simulink model "draft7"  (R2023a)
settings: Solver=VariableStepAuto  StartTime=0.0  StopTime=10  FixedStep=0.0001  MaxStep=0.1  RelTol=1e-3  AbsTol=1e-3  EnableMultiTasking=on
model workspace (MAT data in the model file):
  C_Gimbal = 0.1
  C_IAP = 0.01
  IAP_Pa = 0
  K_Gimbal = 0
  K_IAP = 10
  LeftAbdominalMuscleForce = 0
  LeftBackMuscleForce = 0
  LeftTransverse1MuscleForce = 0
  LeftTransverse2MuscleForce = 0
  Moment_AR = 0
  Moment_FE = 0
  Moment_LB = 0
  RightAbdominalMuscleForce = 0
  RightBackMuscleForce = 0
  RightTransverse1MuscleForce = 0
  RightTransverse2MuscleForce = 0
  a = 1
  b = 1
undefined symbols (not defined in the file): X, Y, Z
libraries: sm_lib x279, nesl_utility x233, simulink_extras x33, checkpacklib x3, simulink x1
(part 7 of 7)

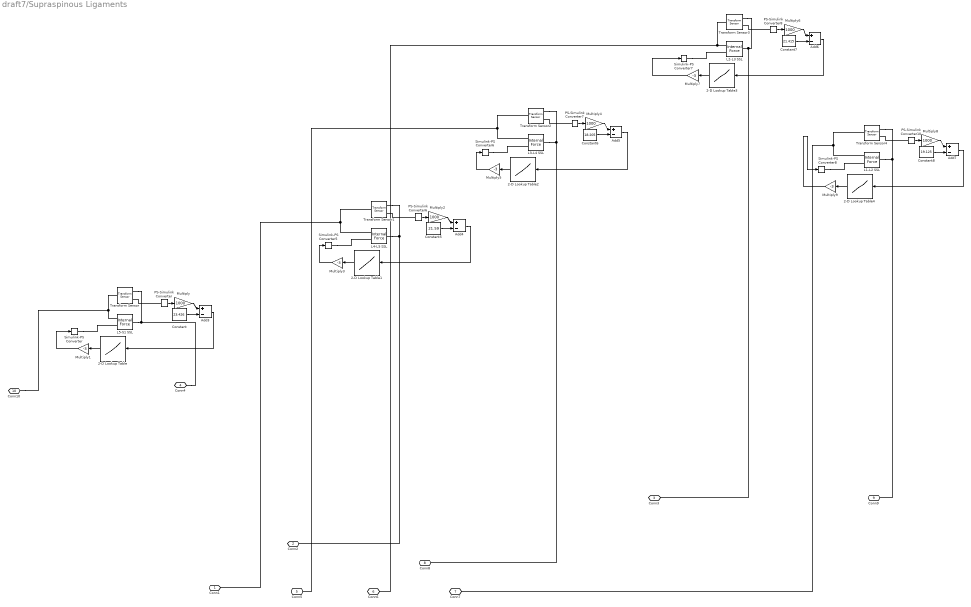
== system draft7/Supraspinous Ligaments ==
  2-D Lookup Table : Lookup_n-D  NumberOfTableDimensions=1  BreakpointsForDimension1=[0;0.272;4.08;5.984;7.888]  BreakpointsForDimension2=[1:3]  Table=[0;0;8.4;21;84]  InternalRulePriority=Speed  RndMeth=Simplest
  2-D Lookup Table1 : Lookup_n-D  NumberOfTableDimensions=1  BreakpointsForDimension1=[0;0.223;3.345;4.906;6.467]  BreakpointsForDimension2=[1:3]  Table=[0;0;8.4;21;84]  InternalRulePriority=Speed  RndMeth=Simplest
  2-D Lookup Table2 : Lookup_n-D  NumberOfTableDimensions=1  BreakpointsForDimension1=[0;0.194;2.91;4.268;5.626]  BreakpointsForDimension2=[1:3]  Table=[0;0;8.4;21;84]  InternalRulePriority=Speed  RndMeth=Simplest
  2-D Lookup Table3 : Lookup_n-D  NumberOfTableDimensions=1  BreakpointsForDimension1=[0;0.268;4.02;5.896;7.772]  BreakpointsForDimension2=[1:3]  Table=[0;0;8.4;21;84]  InternalRulePriority=Speed  RndMeth=Simplest
  2-D Lookup Table4 : Lookup_n-D  NumberOfTableDimensions=1  BreakpointsForDimension1=[0;0.223;3.345;4.906;6.467]  BreakpointsForDimension2=[1:3]  Table=[0;0;8.4;21;84]  InternalRulePriority=Speed  RndMeth=Simplest
  Add{3..7} (5 alike) : Sum  Inputs=+-
  Constant : Constant  Value=23.426
  Constant5 : Constant  Value=21.59
  Constant6 : Constant  Value=18.205
  Constant7 : Constant  Value=21.415
  Constant8 : Constant  Value=19.125
  L1-L2 SSL : sm_lib/Forces and Torques/Internal Force
  L2-L3 SSL : sm_lib/Forces and Torques/Internal Force
  L3-L4 SSL : sm_lib/Forces and Torques/Internal Force
  L4-L5 SSL : sm_lib/Forces and Torques/Internal Force
  L5-S1 SSL : sm_lib/Forces and Torques/Internal Force
  Multiply{,2,4,6,8} (5 alike) : Gain  Gain=1000
  Multiply{1,3,5,7,9} (5 alike) : Gain  Gain=-3
  PS-Simulink Converter{,6..8,10} (5 alike) : nesl_utility/PS-Simulink Converter  PhysicalDomain=network_engine_domain  SubClassName=ps_output  LeftPortType=input  RightPortType=output  PseudoPeriodic=off  Frequencies=[]  VectorFormat=inherit  Unit=inherit  AffineConversion=off
  Simulink-PS Converter{,5..8} (5 alike) : nesl_utility/Simulink-PS Converter  PhysicalDomain=network_engine_domain  SubClassName=ps_input  LeftPortType=input  RightPortType=output  PseudoPeriodic=off  Frequencies=[]  NoiseDistribution=none  NoiseParameters=[]  Unit=1  AffineConversion=off  FilteringAndDerivatives=provide  SimscapeFilterOrder=1  InputFilterTimeConstant=0.001  UdotUserProvided=0
  Transform Sensor{,1..4} (5 alike) : sm_lib/Frames and Transforms/Transform Sensor  MeasurementFrame=World  RotationSequence=XYX  SenseAngle=off  SenseAxis=off  SenseQ=off  SenseR=off  SenseRotationSequence=off  SenseOmegaX=off  SenseOmegaY=off  SenseOmegaZ=off  SenseQDot=off  SenseRDot=off  SenseRotationSequenceDot=off  SenseAlphaX=off  SenseAlphaY=off  SenseAlphaZ=off  SenseQDDot=off  SenseRDDot=off  SenseX=off  SenseY=off  SenseZ=off  SenseRad=off  SenseAzim=off  SenseDist=on  SenseInc=off  SenseXDot=off  SenseYDot=off  SenseZDot=off  SenseRadDot=off  SenseAzimDot=off  SenseDistDot=off  SenseIncDot=off  SenseXDDot=off  SenseYDDot=off  SenseZDDot=off  SenseRadDDot=off  SenseAzimDDot=off  SenseDistDDot=off  SenseIncDDot=off
  Conn1 : PMIOPort  Side=Left
  Conn2 : PMIOPort  Port=2  Side=Left
  Conn3 : PMIOPort  Port=3  Side=Left
  Conn4 : PMIOPort  Port=4  Side=Left
  Conn5 : PMIOPort  Port=5  Side=Left
  Conn6 : PMIOPort  Port=6  Side=Left
  Conn7 : PMIOPort  Port=7  Side=Left
  Conn8 : PMIOPort  Port=8  Side=Left
  Conn9 : PMIOPort  Port=9  Side=Left
  Conn10 : PMIOPort  Port=10  Side=Left
  wires:
  Constant6/1 -> Add5/2
  Add6/1 -> 2-D Lookup Table3/1
  PS-Simulink Converter10/1 -> Multiply8/1
  Add4/1 -> 2-D Lookup Table1/1
  Multiply1/1 -> Simulink-PS Converter/1
  Multiply/1 -> Add3/1
  Multiply7/1 -> Simulink-PS Converter7/1
  Multiply8/1 -> Add7/1
  2-D Lookup Table3/1 -> Multiply7/1
  Multiply6/1 -> Add6/1
  Add3/1 -> 2-D Lookup Table/1
  2-D Lookup Table2/1 -> Multiply5/1
  Constant5/1 -> Add4/2
  PS-Simulink Converter/1 -> Multiply/1
  Constant/1 -> Add3/2
  2-D Lookup Table/1 -> Multiply1/1
  2-D Lookup Table4/1 -> Multiply9/1
  Multiply2/1 -> Add4/1
  Add7/1 -> 2-D Lookup Table4/1
  Multiply3/1 -> Simulink-PS Converter5/1
  Add5/1 -> 2-D Lookup Table2/1
  PS-Simulink Converter8/1 -> Multiply6/1
  Constant7/1 -> Add6/2
  Multiply9/1 -> Simulink-PS Converter8/1
  Constant8/1 -> Add7/2
  2-D Lookup Table1/1 -> Multiply3/1
  Multiply5/1 -> Simulink-PS Converter6/1
  PS-Simulink Converter6/1 -> Multiply2/1
  Multiply4/1 -> Add5/1
  PS-Simulink Converter7/1 -> Multiply4/1
  connections:
  L5-S1 SSL/LConn1 -- Conn10/RConn1 -- Transform Sensor/LConn1
  Simulink-PS Converter8/RConn1 -- L1-L2 SSL/LConn2
  L4-L5 SSL/LConn1 -- Conn1/RConn1 -- Transform Sensor1/LConn1
  L1-L2 SSL/LConn1 -- Conn7/RConn1 -- Transform Sensor4/LConn1
  Simulink-PS Converter/RConn1 -- L5-S1 SSL/LConn2
  PS-Simulink Converter6/LConn1 -- Transform Sensor1/RConn2
  L4-L5 SSL/RConn1 -- Transform Sensor1/RConn1 -- Conn2/RConn1
  PS-Simulink Converter/LConn1 -- Transform Sensor/RConn2
  L5-S1 SSL/RConn1 -- Conn4/RConn1 -- Transform Sensor/RConn1
  L3-L4 SSL/LConn1 -- Conn5/RConn1 -- Transform Sensor2/LConn1
  PS-Simulink Converter8/LConn1 -- Transform Sensor3/RConn2
  PS-Simulink Converter10/LConn1 -- Transform Sensor4/RConn2
  L2-L3 SSL/RConn1 -- Conn3/RConn1 -- Transform Sensor3/RConn1
  PS-Simulink Converter7/LConn1 -- Transform Sensor2/RConn2
  L1-L2 SSL/RConn1 -- Conn9/RConn1 -- Transform Sensor4/RConn1
  L2-L3 SSL/LConn1 -- Conn6/RConn1 -- Transform Sensor3/LConn1
  Transform Sensor2/RConn1 -- Conn8/RConn1 -- L3-L4 SSL/RConn1
  Simulink-PS Converter7/RConn1 -- L2-L3 SSL/LConn2
  Simulink-PS Converter5/RConn1 -- L4-L5 SSL/LConn2
  Simulink-PS Converter6/RConn1 -- L3-L4 SSL/LConn2

== system draft7/L1/AR torque feedback L4 ==
  Constant : Constant  Value=0.7
  Constant1 : Constant  Value=0.7
  Gain5 : Gain  Gain=-1
  PS-Simulink Converter9 : nesl_utility/PS-Simulink Converter  PhysicalDomain=network_engine_domain  SubClassName=ps_output  LeftPortType=input  RightPortType=output  PseudoPeriodic=off  Frequencies=[]  VectorFormat=1-D array  Unit=inherit  AffineConversion=off
  Radians to Degrees : simulink_extras/Transformations/Radians to Degrees
  Simulink-PS Converter6 : nesl_utility/Simulink-PS Converter  PhysicalDomain=network_engine_domain  SubClassName=ps_input  LeftPortType=input  RightPortType=output  PseudoPeriodic=off  Frequencies=[]  NoiseDistribution=none  NoiseParameters=[]  Unit=1  AffineConversion=off  FilteringAndDerivatives=provide  SimscapeFilterOrder=1  InputFilterTimeConstant=0.001  UdotUserProvided=0
  peacewise torque profile5 : MATLAB Function  TreatAsAtomicUnit=on
  AR rot : PMIOPort  Side=Left
  AR torque : PMIOPort  Port=2  Side=Right
  wires:
  PS-Simulink Converter9/1 -> Radians to Degrees/1
  peacewise torque profile5/1(torque) -> Gain5/1
  Gain5/1 -> Simulink-PS Converter6/1
  Radians to Degrees/1 -> peacewise torque profile5/1(u)
  Constant/1 -> peacewise torque profile5/2(a)
  Constant1/1 -> peacewise torque profile5/3(b)
  connections:
  PS-Simulink Converter9/LConn1 -- AR rot/RConn1
  AR torque/RConn1 -- Simulink-PS Converter6/RConn1

== system draft7/L1/FE torque feedback L4 ==
  Constant : Constant  Value=a
  Constant1 : Constant  Value=b
  Gain1 : Gain  Gain=-1
  Gain7 : Gain
  PS-Simulink Converter5 : nesl_utility/PS-Simulink Converter  PhysicalDomain=network_engine_domain  SubClassName=ps_output  LeftPortType=input  RightPortType=output  PseudoPeriodic=off  Frequencies=[]  VectorFormat=1-D array  Unit=inherit  AffineConversion=off
  Radians to Degrees : simulink_extras/Transformations/Radians to Degrees
  Simulink-PS Converter4 : nesl_utility/Simulink-PS Converter  PhysicalDomain=network_engine_domain  SubClassName=ps_input  LeftPortType=input  RightPortType=output  PseudoPeriodic=off  Frequencies=[]  NoiseDistribution=none  NoiseParameters=[]  Unit=1  AffineConversion=off  FilteringAndDerivatives=provide  SimscapeFilterOrder=1  InputFilterTimeConstant=0.001  UdotUserProvided=0
  peacewise torque profile1 : MATLAB Function  TreatAsAtomicUnit=on
  FE rot : PMIOPort  Side=Left
  FE torque : PMIOPort  Port=2  Side=Right
  wires:
  PS-Simulink Converter5/1 -> Radians to Degrees/1
  peacewise torque profile1/1(torque) -> Gain7/1
  Gain7/1 -> Simulink-PS Converter4/1
  Radians to Degrees/1 -> Gain1/1
  Gain1/1 -> peacewise torque profile1/1(u)
  Constant/1 -> peacewise torque profile1/2(a)
  Constant1/1 -> peacewise torque profile1/3(b)
  connections:
  FE rot/RConn1 -- PS-Simulink Converter5/LConn1
  FE torque/RConn1 -- Simulink-PS Converter4/RConn1

== system draft7/L1/LB torque feedback L4 ==
  Constant : Constant  Value=a
  Constant1 : Constant  Value=b
  Gain4 : Gain  Gain=-1
  PS-Simulink Converter8 : nesl_utility/PS-Simulink Converter  PhysicalDomain=network_engine_domain  SubClassName=ps_output  LeftPortType=input  RightPortType=output  PseudoPeriodic=off  Frequencies=[]  VectorFormat=1-D array  Unit=inherit  AffineConversion=off
  Radians to Degrees : simulink_extras/Transformations/Radians to Degrees
  Simulink-PS Converter5 : nesl_utility/Simulink-PS Converter  PhysicalDomain=network_engine_domain  SubClassName=ps_input  LeftPortType=input  RightPortType=output  PseudoPeriodic=off  Frequencies=[]  NoiseDistribution=none  NoiseParameters=[]  Unit=1  AffineConversion=off  FilteringAndDerivatives=provide  SimscapeFilterOrder=1  InputFilterTimeConstant=0.001  UdotUserProvided=0
  peacewise torque profile4 : MATLAB Function  TreatAsAtomicUnit=on
  LB rot : PMIOPort  Side=Left
  LB torque : PMIOPort  Port=2  Side=Right
  wires:
  Gain4/1 -> Simulink-PS Converter5/1
  PS-Simulink Converter8/1 -> Radians to Degrees/1
  peacewise torque profile4/1(torque) -> Gain4/1
  Constant/1 -> peacewise torque profile4/2(a)
  Constant1/1 -> peacewise torque profile4/3(b)
  Radians to Degrees/1 -> peacewise torque profile4/1(u)
  connections:
  Simulink-PS Converter5/RConn1 -- LB torque/RConn1
  LB rot/RConn1 -- PS-Simulink Converter8/LConn1

== system draft7/L2/AR torque feedback L4 ==
  Constant : Constant  Value=0.7
  Constant1 : Constant  Value=0.7
  Gain5 : Gain  Gain=-1
  PS-Simulink Converter9 : nesl_utility/PS-Simulink Converter  PhysicalDomain=network_engine_domain  SubClassName=ps_output  LeftPortType=input  RightPortType=output  PseudoPeriodic=off  Frequencies=[]  VectorFormat=1-D array  Unit=inherit  AffineConversion=off
  Radians to Degrees : simulink_extras/Transformations/Radians to Degrees
  Simulink-PS Converter6 : nesl_utility/Simulink-PS Converter  PhysicalDomain=network_engine_domain  SubClassName=ps_input  LeftPortType=input  RightPortType=output  PseudoPeriodic=off  Frequencies=[]  NoiseDistribution=none  NoiseParameters=[]  Unit=1  AffineConversion=off  FilteringAndDerivatives=provide  SimscapeFilterOrder=1  InputFilterTimeConstant=0.001  UdotUserProvided=0
  peacewise torque profile5 : MATLAB Function  TreatAsAtomicUnit=on
  AR rot : PMIOPort  Side=Left
  AR torque : PMIOPort  Port=2  Side=Right
  wires:
  Gain5/1 -> Simulink-PS Converter6/1
  peacewise torque profile5/1(torque) -> Gain5/1
  PS-Simulink Converter9/1 -> Radians to Degrees/1
  Radians to Degrees/1 -> peacewise torque profile5/1(u)
  Constant/1 -> peacewise torque profile5/2(a)
  Constant1/1 -> peacewise torque profile5/3(b)
  connections:
  AR torque/RConn1 -- Simulink-PS Converter6/RConn1
  PS-Simulink Converter9/LConn1 -- AR rot/RConn1

== system draft7/L2/FE torque feedback L4 ==
  Constant : Constant  Value=a
  Constant1 : Constant  Value=b
  Gain1 : Gain  Gain=-1
  Gain7 : Gain
  PS-Simulink Converter5 : nesl_utility/PS-Simulink Converter  PhysicalDomain=network_engine_domain  SubClassName=ps_output  LeftPortType=input  RightPortType=output  PseudoPeriodic=off  Frequencies=[]  VectorFormat=1-D array  Unit=inherit  AffineConversion=off
  Radians to Degrees : simulink_extras/Transformations/Radians to Degrees
  Simulink-PS Converter4 : nesl_utility/Simulink-PS Converter  PhysicalDomain=network_engine_domain  SubClassName=ps_input  LeftPortType=input  RightPortType=output  PseudoPeriodic=off  Frequencies=[]  NoiseDistribution=none  NoiseParameters=[]  Unit=1  AffineConversion=off  FilteringAndDerivatives=provide  SimscapeFilterOrder=1  InputFilterTimeConstant=0.001  UdotUserProvided=0
  peacewise torque profile1 : MATLAB Function  TreatAsAtomicUnit=on
  FE rot : PMIOPort  Side=Left
  FE torque : PMIOPort  Port=2  Side=Right
  wires:
  Gain7/1 -> Simulink-PS Converter4/1
  peacewise torque profile1/1(torque) -> Gain7/1
  Radians to Degrees/1 -> Gain1/1
  PS-Simulink Converter5/1 -> Radians to Degrees/1
  Constant/1 -> peacewise torque profile1/2(a)
  Constant1/1 -> peacewise torque profile1/3(b)
  Gain1/1 -> peacewise torque profile1/1(u)
  connections:
  FE torque/RConn1 -- Simulink-PS Converter4/RConn1
  FE rot/RConn1 -- PS-Simulink Converter5/LConn1

== system draft7/L2/LB torque feedback L4 ==
  Constant : Constant  Value=a
  Constant1 : Constant  Value=b
  Gain4 : Gain  Gain=-1
  PS-Simulink Converter8 : nesl_utility/PS-Simulink Converter  PhysicalDomain=network_engine_domain  SubClassName=ps_output  LeftPortType=input  RightPortType=output  PseudoPeriodic=off  Frequencies=[]  VectorFormat=1-D array  Unit=inherit  AffineConversion=off
  Radians to Degrees : simulink_extras/Transformations/Radians to Degrees
  Simulink-PS Converter5 : nesl_utility/Simulink-PS Converter  PhysicalDomain=network_engine_domain  SubClassName=ps_input  LeftPortType=input  RightPortType=output  PseudoPeriodic=off  Frequencies=[]  NoiseDistribution=none  NoiseParameters=[]  Unit=1  AffineConversion=off  FilteringAndDerivatives=provide  SimscapeFilterOrder=1  InputFilterTimeConstant=0.001  UdotUserProvided=0
  peacewise torque profile4 : MATLAB Function  TreatAsAtomicUnit=on
  LB rot : PMIOPort  Side=Left
  LB torque : PMIOPort  Port=2  Side=Right
  wires:
  peacewise torque profile4/1(torque) -> Gain4/1
  PS-Simulink Converter8/1 -> Radians to Degrees/1
  Gain4/1 -> Simulink-PS Converter5/1
  Constant/1 -> peacewise torque profile4/2(a)
  Constant1/1 -> peacewise torque profile4/3(b)
  Radians to Degrees/1 -> peacewise torque profile4/1(u)
  connections:
  LB rot/RConn1 -- PS-Simulink Converter8/LConn1
  Simulink-PS Converter5/RConn1 -- LB torque/RConn1

== system draft7/L3/AR torque feedback L4 ==
  Constant : Constant  Value=0.7
  Constant1 : Constant  Value=0.7
  Gain5 : Gain  Gain=-1
  PS-Simulink Converter9 : nesl_utility/PS-Simulink Converter  PhysicalDomain=network_engine_domain  SubClassName=ps_output  LeftPortType=input  RightPortType=output  PseudoPeriodic=off  Frequencies=[]  VectorFormat=1-D array  Unit=inherit  AffineConversion=off
  Radians to Degrees : simulink_extras/Transformations/Radians to Degrees
  Simulink-PS Converter6 : nesl_utility/Simulink-PS Converter  PhysicalDomain=network_engine_domain  SubClassName=ps_input  LeftPortType=input  RightPortType=output  PseudoPeriodic=off  Frequencies=[]  NoiseDistribution=none  NoiseParameters=[]  Unit=1  AffineConversion=off  FilteringAndDerivatives=provide  SimscapeFilterOrder=1  InputFilterTimeConstant=0.001  UdotUserProvided=0
  peacewise torque profile5 : MATLAB Function  TreatAsAtomicUnit=on
  AR rot : PMIOPort  Side=Left
  AR torque : PMIOPort  Port=2  Side=Right
  wires:
  peacewise torque profile5/1(torque) -> Gain5/1
  Gain5/1 -> Simulink-PS Converter6/1
  PS-Simulink Converter9/1 -> Radians to Degrees/1
  Radians to Degrees/1 -> peacewise torque profile5/1(u)
  Constant/1 -> peacewise torque profile5/2(a)
  Constant1/1 -> peacewise torque profile5/3(b)
  connections:
  PS-Simulink Converter9/LConn1 -- AR rot/RConn1
  AR torque/RConn1 -- Simulink-PS Converter6/RConn1

== system draft7/L3/FE torque feedback L4 ==
  Constant : Constant  Value=a
  Constant1 : Constant  Value=b
  Gain1 : Gain  Gain=-1
  Gain7 : Gain
  PS-Simulink Converter5 : nesl_utility/PS-Simulink Converter  PhysicalDomain=network_engine_domain  SubClassName=ps_output  LeftPortType=input  RightPortType=output  PseudoPeriodic=off  Frequencies=[]  VectorFormat=1-D array  Unit=inherit  AffineConversion=off
  Radians to Degrees : simulink_extras/Transformations/Radians to Degrees
  Simulink-PS Converter4 : nesl_utility/Simulink-PS Converter  PhysicalDomain=network_engine_domain  SubClassName=ps_input  LeftPortType=input  RightPortType=output  PseudoPeriodic=off  Frequencies=[]  NoiseDistribution=none  NoiseParameters=[]  Unit=1  AffineConversion=off  FilteringAndDerivatives=provide  SimscapeFilterOrder=1  InputFilterTimeConstant=0.001  UdotUserProvided=0
  peacewise torque profile1 : MATLAB Function  TreatAsAtomicUnit=on
  FE rot : PMIOPort  Side=Left
  FE torque : PMIOPort  Port=2  Side=Right
  wires:
  peacewise torque profile1/1(torque) -> Gain7/1
  Gain7/1 -> Simulink-PS Converter4/1
  Radians to Degrees/1 -> Gain1/1
  PS-Simulink Converter5/1 -> Radians to Degrees/1
  Constant/1 -> peacewise torque profile1/2(a)
  Constant1/1 -> peacewise torque profile1/3(b)
  Gain1/1 -> peacewise torque profile1/1(u)
  connections:
  FE rot/RConn1 -- PS-Simulink Converter5/LConn1
  FE torque/RConn1 -- Simulink-PS Converter4/RConn1

== system draft7/L3/LB torque feedback L4 ==
  Constant : Constant  Value=a
  Constant1 : Constant  Value=b
  Gain4 : Gain  Gain=-1
  PS-Simulink Converter8 : nesl_utility/PS-Simulink Converter  PhysicalDomain=network_engine_domain  SubClassName=ps_output  LeftPortType=input  RightPortType=output  PseudoPeriodic=off  Frequencies=[]  VectorFormat=1-D array  Unit=inherit  AffineConversion=off
  Radians to Degrees : simulink_extras/Transformations/Radians to Degrees
  Simulink-PS Converter5 : nesl_utility/Simulink-PS Converter  PhysicalDomain=network_engine_domain  SubClassName=ps_input  LeftPortType=input  RightPortType=output  PseudoPeriodic=off  Frequencies=[]  NoiseDistribution=none  NoiseParameters=[]  Unit=1  AffineConversion=off  FilteringAndDerivatives=provide  SimscapeFilterOrder=1  InputFilterTimeConstant=0.001  UdotUserProvided=0
  peacewise torque profile4 : MATLAB Function  TreatAsAtomicUnit=on
  LB rot : PMIOPort  Side=Left
  LB torque : PMIOPort  Port=2  Side=Right
  wires:
  Gain4/1 -> Simulink-PS Converter5/1
  PS-Simulink Converter8/1 -> Radians to Degrees/1
  peacewise torque profile4/1(torque) -> Gain4/1
  Constant/1 -> peacewise torque profile4/2(a)
  Constant1/1 -> peacewise torque profile4/3(b)
  Radians to Degrees/1 -> peacewise torque profile4/1(u)
  connections:
  Simulink-PS Converter5/RConn1 -- LB torque/RConn1
  LB rot/RConn1 -- PS-Simulink Converter8/LConn1

== system draft7/L4/AR torque feedback L4 ==
  Constant : Constant  Value=0.7
  Constant1 : Constant  Value=0.7
  Gain5 : Gain  Gain=-1
  PS-Simulink Converter9 : nesl_utility/PS-Simulink Converter  PhysicalDomain=network_engine_domain  SubClassName=ps_output  LeftPortType=input  RightPortType=output  PseudoPeriodic=off  Frequencies=[]  VectorFormat=1-D array  Unit=inherit  AffineConversion=off
  Radians to Degrees : simulink_extras/Transformations/Radians to Degrees
  Simulink-PS Converter6 : nesl_utility/Simulink-PS Converter  PhysicalDomain=network_engine_domain  SubClassName=ps_input  LeftPortType=input  RightPortType=output  PseudoPeriodic=off  Frequencies=[]  NoiseDistribution=none  NoiseParameters=[]  Unit=1  AffineConversion=off  FilteringAndDerivatives=provide  SimscapeFilterOrder=1  InputFilterTimeConstant=0.001  UdotUserProvided=0
  peacewise torque profile5 : MATLAB Function  TreatAsAtomicUnit=on
  AR rot : PMIOPort  Side=Left
  AR torque : PMIOPort  Port=2  Side=Right
  wires:
  Gain5/1 -> Simulink-PS Converter6/1
  peacewise torque profile5/1(torque) -> Gain5/1
  PS-Simulink Converter9/1 -> Radians to Degrees/1
  Radians to Degrees/1 -> peacewise torque profile5/1(u)
  Constant/1 -> peacewise torque profile5/2(a)
  Constant1/1 -> peacewise torque profile5/3(b)
  connections:
  AR torque/RConn1 -- Simulink-PS Converter6/RConn1
  PS-Simulink Converter9/LConn1 -- AR rot/RConn1

== system draft7/L4/FE torque feedback L4 ==
  Constant : Constant  Value=a
  Constant1 : Constant  Value=b
  Gain1 : Gain  Gain=-1
  Gain7 : Gain
  PS-Simulink Converter5 : nesl_utility/PS-Simulink Converter  PhysicalDomain=network_engine_domain  SubClassName=ps_output  LeftPortType=input  RightPortType=output  PseudoPeriodic=off  Frequencies=[]  VectorFormat=1-D array  Unit=inherit  AffineConversion=off
  Radians to Degrees : simulink_extras/Transformations/Radians to Degrees
  Scope : Scope  NumInputPorts=2
  Simulink-PS Converter4 : nesl_utility/Simulink-PS Converter  PhysicalDomain=network_engine_domain  SubClassName=ps_input  LeftPortType=input  RightPortType=output  PseudoPeriodic=off  Frequencies=[]  NoiseDistribution=none  NoiseParameters=[]  Unit=1  AffineConversion=off  FilteringAndDerivatives=provide  SimscapeFilterOrder=1  InputFilterTimeConstant=0.001  UdotUserProvided=0
  peacewise torque profile1 : MATLAB Function  TreatAsAtomicUnit=on
  FE rot : PMIOPort  Side=Left
  FE torque : PMIOPort  Port=2  Side=Right
  wires:
  Gain7/1 -> Scope/2, Simulink-PS Converter4/1
  peacewise torque profile1/1(torque) -> Gain7/1
  Radians to Degrees/1 -> Gain1/1
  PS-Simulink Converter5/1 -> Radians to Degrees/1
  Constant/1 -> peacewise torque profile1/2(a)
  Constant1/1 -> peacewise torque profile1/3(b)
  Gain1/1 -> Scope/1, peacewise torque profile1/1(u)
  connections:
  FE torque/RConn1 -- Simulink-PS Converter4/RConn1
  FE rot/RConn1 -- PS-Simulink Converter5/LConn1

== system draft7/L4/LB torque feedback L4 ==
  Constant : Constant  Value=a
  Constant1 : Constant  Value=b
  Gain4 : Gain  Gain=-1
  PS-Simulink Converter8 : nesl_utility/PS-Simulink Converter  PhysicalDomain=network_engine_domain  SubClassName=ps_output  LeftPortType=input  RightPortType=output  PseudoPeriodic=off  Frequencies=[]  VectorFormat=1-D array  Unit=inherit  AffineConversion=off
  Radians to Degrees : simulink_extras/Transformations/Radians to Degrees
  Simulink-PS Converter5 : nesl_utility/Simulink-PS Converter  PhysicalDomain=network_engine_domain  SubClassName=ps_input  LeftPortType=input  RightPortType=output  PseudoPeriodic=off  Frequencies=[]  NoiseDistribution=none  NoiseParameters=[]  Unit=1  AffineConversion=off  FilteringAndDerivatives=provide  SimscapeFilterOrder=1  InputFilterTimeConstant=0.001  UdotUserProvided=0
  peacewise torque profile4 : MATLAB Function  TreatAsAtomicUnit=on
  LB rot : PMIOPort  Side=Left
  LB torque : PMIOPort  Port=2  Side=Right
  wires:
  peacewise torque profile4/1(torque) -> Gain4/1
  PS-Simulink Converter8/1 -> Radians to Degrees/1
  Gain4/1 -> Simulink-PS Converter5/1
  Constant/1 -> peacewise torque profile4/2(a)
  Constant1/1 -> peacewise torque profile4/3(b)
  Radians to Degrees/1 -> peacewise torque profile4/1(u)
  connections:
  LB rot/RConn1 -- PS-Simulink Converter8/LConn1
  Simulink-PS Converter5/RConn1 -- LB torque/RConn1

== system draft7/L5/AR torque feedback L5 ==
  Constant : Constant  Value=0.7
  Constant1 : Constant  Value=0.7
  Gain2 : Gain  Gain=-1
  PS-Simulink Converter3 : nesl_utility/PS-Simulink Converter  PhysicalDomain=network_engine_domain  SubClassName=ps_output  LeftPortType=input  RightPortType=output  PseudoPeriodic=off  Frequencies=[]  VectorFormat=1-D array  Unit=inherit  AffineConversion=off
  Radians to Degrees : simulink_extras/Transformations/Radians to Degrees
  Simulink-PS Converter2 : nesl_utility/Simulink-PS Converter  PhysicalDomain=network_engine_domain  SubClassName=ps_input  LeftPortType=input  RightPortType=output  PseudoPeriodic=off  Frequencies=[]  NoiseDistribution=none  NoiseParameters=[]  Unit=1  AffineConversion=off  FilteringAndDerivatives=provide  SimscapeFilterOrder=1  InputFilterTimeConstant=0.001  UdotUserProvided=0
  peacewise torque profile3 : MATLAB Function  TreatAsAtomicUnit=on
  AR rot : PMIOPort  Side=Left
  AR torque : PMIOPort  Port=2  Side=Right
  wires:
  peacewise torque profile3/1(torque) -> Gain2/1
  Gain2/1 -> Simulink-PS Converter2/1
  PS-Simulink Converter3/1 -> Radians to Degrees/1
  Radians to Degrees/1 -> peacewise torque profile3/1(u)
  Constant/1 -> peacewise torque profile3/2(a)
  Constant1/1 -> peacewise torque profile3/3(b)
  connections:
  AR torque/RConn1 -- Simulink-PS Converter2/RConn1
  PS-Simulink Converter3/LConn1 -- AR rot/RConn1

== system draft7/L5/FE torque feedback L5 ==
  Constant : Constant  Value=a
  Constant1 : Constant  Value=b
  Gain1 : Gain  Gain=-1
  Gain6 : Gain
  PS-Simulink Converter : nesl_utility/PS-Simulink Converter  PhysicalDomain=network_engine_domain  SubClassName=ps_output  LeftPortType=input  RightPortType=output  PseudoPeriodic=off  Frequencies=[]  VectorFormat=inherit  Unit=inherit  AffineConversion=off
  Radians to Degrees : simulink_extras/Transformations/Radians to Degrees
  Scope : Scope  NumInputPorts=2
  Simulink-PS Converter3 : nesl_utility/Simulink-PS Converter  PhysicalDomain=network_engine_domain  SubClassName=ps_input  LeftPortType=input  RightPortType=output  PseudoPeriodic=off  Frequencies=[]  NoiseDistribution=none  NoiseParameters=[]  Unit=1  AffineConversion=off  FilteringAndDerivatives=provide  SimscapeFilterOrder=1  InputFilterTimeConstant=0.001  UdotUserProvided=0
  XY Graph : Record  FileSettingsInternal="{\"entries\":[{\"content\":{\"excelSettings\":{\"content\":{},\"type\":\"Streamout.ExcelSettings\"}},\"type\":\"Streamout.FileSettingStorage\",\"uuid\":\"bb662e76-cdb6-4b93-b149-242342cb3116\"}],\"packageUris\":[\"http://schema.mathworks.com/mf0/streamout_blocks/R2020a\"],\"version\":\"1.0\"}"  Layout=[1 1]  SignalsInternal="{\"entries\":[{\"content\":{\"signals\":[{\"content\":{\"blockPath\":[\"draft7/L5/FE torque feedback L5/XY Graph\"],\"dimensions\":[1],\"domain\":\"draft7/L5/FE torque feedback L5/XY Graph\",\"lineColor\":\"#0072bd\",\"port\":1,\"sid\":[\"\"],\"signalID\":291,\"signalName\":\"moment\"},\"type\":\"RecordBlkView.Signal\",\"uuid\":\"f33ae304-b7fa-4d6f-a128-695caf737a37\"},{\"content\":{\"blockPath\":[\"draft7/L5/FE torque feedback L5/XY Graph\"],\"dimensions\":[1,1],\"domain\":\"draft7/L5/FE torque feedback L5/XY Graph\",\"lineColor\":\"#d95319\",\"port\":2,\"sid\":[\"\"],\"signalID\":296,\"signalName\":\"rot\"},\"type\":\"RecordBlkView.Signal\",\"uuid\":\"2c48db8a-27da-43a1-9e6c-93f0abff24cf\"}]},\"type\":\"RecordBlkView.InputSignals\",\"uuid\":\"0e2f0ee8-3720-49e6-9af3-fa45cfe012d6\"}],\"packageUris\":[\"http://schema.mathworks.com/mf0/streamout_blocks/R2020a\"],\"version\":\"1.0\"}"  VisualizationBindings="{\"xyplotplugin\":{\"info\":[{\"series\":[],\"subplotID\":1}]}}"  CompatibilityTag=XY
  peacewise torque profile (+- 15 deg) : MATLAB Function  TreatAsAtomicUnit=on
  FE torque : PMIOPort  Side=Right
  FE rot : PMIOPort  Port=2  Side=Left
  wires:
  Gain6/1 -> XY Graph/1, Scope/1, Simulink-PS Converter3/1  "moment"
  peacewise torque profile (+- 15 deg)/1(torque) -> Gain6/1
  Radians to Degrees/1 -> Gain1/1
  PS-Simulink Converter/1 -> Radians to Degrees/1
  Constant/1 -> peacewise torque profile (+- 15 deg)/2(a)
  Constant1/1 -> peacewise torque profile (+- 15 deg)/3(b)
  Gain1/1 -> XY Graph/2, Scope/2, peacewise torque profile (+- 15 deg)/1(u)  "rot"
  connections:
  FE rot/RConn1 -- PS-Simulink Converter/LConn1
  Simulink-PS Converter3/RConn1 -- FE torque/RConn1

== system draft7/L5/LB torque feedback L5 ==
  Constant : Constant  Value=a
  Constant1 : Constant  Value=b
  Gain1 : Gain  Gain=-1
  PS-Simulink Converter2 : nesl_utility/PS-Simulink Converter  PhysicalDomain=network_engine_domain  SubClassName=ps_output  LeftPortType=input  RightPortType=output  PseudoPeriodic=off  Frequencies=[]  VectorFormat=1-D array  Unit=inherit  AffineConversion=off
  Radians to Degrees : simulink_extras/Transformations/Radians to Degrees
  Simulink-PS Converter1 : nesl_utility/Simulink-PS Converter  PhysicalDomain=network_engine_domain  SubClassName=ps_input  LeftPortType=input  RightPortType=output  PseudoPeriodic=off  Frequencies=[]  NoiseDistribution=none  NoiseParameters=[]  Unit=1  AffineConversion=off  FilteringAndDerivatives=provide  SimscapeFilterOrder=1  InputFilterTimeConstant=0.001  UdotUserProvided=0
  peacewise torque profile2 : MATLAB Function  TreatAsAtomicUnit=on
  LB rot : PMIOPort  Side=Left
  LB torque : PMIOPort  Port=2  Side=Right
  wires:
  Gain1/1 -> Simulink-PS Converter1/1
  PS-Simulink Converter2/1 -> Radians to Degrees/1
  peacewise torque profile2/1(torque) -> Gain1/1
  Constant/1 -> peacewise torque profile2/2(a)
  Constant1/1 -> peacewise torque profile2/3(b)
  Radians to Degrees/1 -> peacewise torque profile2/1(u)
  connections:
  LB rot/RConn1 -- PS-Simulink Converter2/LConn1
  Simulink-PS Converter1/RConn1 -- LB torque/RConn1

== matlab function draft7/L2/FE torque feedback L4/peacewise torque profile1 ==
  data: u input; torque output; a input; b input


function torque = T(u,a,b) % Guan et al logarithmic
    torque = 0;
    if (u >= 0)
     torque= a*(exp(u/8.23)-1)/0.10;

    elseif (u< 0)
     torque= b*(exp(u/-1.31)-1)/(-0.58)   ;
end

% function torque = T(u,a,b) % Rao et al segmental
%     torque = 0;
%     if (u >= 0)
%         torque= (a)*(-0.0042*u^2 + 1.9155*u);
%     elseif (u< 0)
%         torque= (b)*(-0.0042*u^2 + 1.9155*u);
% end

== matlab function draft7/L2/LB torque feedback L4/peacewise torque profile4 ==
  data: u input; torque output; a input; b input
function torque = T(u,a,b)    % Guan et al (nonlinear logarithmic equation mentioned in their paper)
    torque = 0;
    if (u >= 0)
     torque= a*(exp(u/2.13)-1)/0.87;

    elseif (u< 0)
     torque= b*(exp(u/-2.22)-1)/(-0.66)   ;
end

== matlab function draft7/L1/AR torque feedback L4/peacewise torque profile5 ==
  data: u input; torque output; a input; b input
function torque = T(u,a,b)    % Panjabi data fitted into logarithmic equation. Refer validation.xlsx
    torque = 0;
    if (u >= 0)
     torque= a*(exp(u/0.83)-1)/0.35;

    elseif (u < 0)
     torque= b*(exp(u/-0.38)-1)/(-3.18)   ;
end

== matlab function draft7/L1/FE torque feedback L4/peacewise torque profile1 ==
  data: u input; torque output; a input; b input
% function torque = T(u,udot)  % Guan et al logarithmic plus  (RECALCULATED - refer excel)
%     torque = 0;
%     if (u >= 0)
%      torque= (exp(u/8.067)-1)/0.1031   +    0.1*udot;
% 
%     elseif (u < 0)
%      torque= (exp(u/-1.2951)-1)/(-0.5753) +  0.1*udot  ;
% end



function torque = T(u,a,b)  % Guan et al logarithmic  (RECALCULATED - refer excel)
    torque = 0;
    if (u >= 0)
     torque= a*(exp(u/8.067)-1)/0.1031;

    elseif (u < 0)
     torque= b*(exp(u/-1.2951)-1)/(-0.5753)   ;
end


% function torque = T(u,a,b)  % Rao et al segmental
%     torque = 0;
%     if (u >= 0)
%         torque = (a)*(0.0343*u^2 + 1.9989*u);
%     elseif (u < 0)
%         torque = (b)*(0.0343*u^2 + 1.9989*u);
% end

== matlab function draft7/L1/LB torque feedback L4/peacewise torque profile4 ==
  data: u input; torque output; a input; b input
function torque = T(u,a,b)    % Guan et al (RECALCULATED - refer excel)
    torque = 0;
    if (u >= 0)
     torque= a*(exp(u/2.0545)-1)/0.9457;

    elseif (u< 0)
     torque= b*(exp(u/-2.3716)-1)/(-0.5744)   ;
end

== matlab function draft7/L4/FE torque feedback L4/peacewise torque profile1 ==
  data: u input; torque output; a input; b input


function torque = T(u,a,b) % Guan et al logarithmic
    torque = 0;
    if (u >= 0)
     torque= a*(exp(u/3.07)-1)/0.81;

    elseif (u< 0)
     torque= b*(exp(u/-8.14)-1)/(-0.05)   ;
end

% function torque = T(u,a,b) % Rao et al segmental
%     torque = 0;
%     if (u >= 0)
%         torque= (a)*(0.0493*u^2 + 2.2629*u);
%     elseif (u< 0)
%         torque= (b)*(0.0493*u^2 + 2.2629*u);
% end

== matlab function draft7/Muscle Forces/Sum of Square of Forces ==
  data: F1 input; SumofSquareofForces output; F2 input; F3 input; F4 input; F5 input; F6 input; F7 input; F8 input; IAP input
function SumofSquareofForces = fcn(F1,F2,F3,F4,F5,F6,F7,F8,IAP)

SumofSquareofForces = F1^2 + F2^2 + F3^2 + F4^2 + F5^2 + F6^2 +F7^2 + F8^2 + IAP^2;

== matlab function draft7/Sagittaal Kinematics Readings/MATLAB Function ==
  data: y input; angle output; z input
function angle = fcn(y,z)

angle = 90 - (57.2958*atan(z/y));

end

== matlab function draft7/L5/FE torque feedback L5/peacewise torque profile (+- 15 deg) ==
  data: u input; torque output; a input; b input


function torque = T(u,a,b)    % Guan et al (nonlinear logarithmic equation mentioned in their paper)
    torque = 0;
    if (u >= 0)
     torque= a*(exp(u/5.58)-1)/0.59;

    elseif (u< 0)
     torque= b*(exp(u/-4.48)-1)/(-0.33)   ;
end

% function torque = T(u,a,b)    % Rao et al segmental data
%     torque = 0;
%     if (u >= 0)
%         torque= (a)*(0.0348*u^3 + 0.089*u^2 + 1.1837*u);
%     elseif (u< 0)
%         torque= (b)*(0.0348*u^3 + 0.089*u^2 + 1.1837*u);
% end

== matlab function draft7/L5/LB torque feedback L5/peacewise torque profile2 ==
  data: u input; torque output; a input; b input
function torque = T(u,a,b)    % Guan et al (nonlinear logarithmic equation mentioned in their paper)
    torque = 0;
    if (u >= 0)
     torque= a*(exp(u/3.26)-1)/0.49;

    elseif (u < 0)
     torque= b*(exp(u/-4.22)-1)/(-0.29)   ;
end

== matlab function draft7/L5/AR torque feedback L5/peacewise torque profile3 ==
  data: u input; torque output; a input; b input
function torque = T(u,a,b)    % Panjabi data fitted into logarithmic equation. Refer validation.xlsx
    torque = 0;
    if (u >= 0)
     torque= a*(exp(u/1.25)-1)/0.10;

    elseif (u < 0)
     torque= b*(exp(u/-1.05)-1)/(-0.10)   ;
end

== matlab function draft7/L4/LB torque feedback L4/peacewise torque profile4 ==
  data: u input; torque output; a input; b input
function torque = T(u,a,b)    % Guan et al (nonlinear logarithmic equation mentioned in their paper)
    torque = 0;
    if (u >= 0)
     torque= a*(exp(u/1.77)-1)/1.28;

    elseif (u< 0)
     torque= b*(exp(u/-1.44)-1)/(-1.23)   ;
end

== matlab function draft7/L4/AR torque feedback L4/peacewise torque profile5 ==
  data: u input; torque output; a input; b input
function torque = T(u,a,b)    % Panjabi data fitted into logarithmic equation. Refer validation.xlsx
    torque = 0;
    if (u >= 0)
     torque= a*(exp(u/0.73)-1)/0.20;

    elseif (u < 0)
     torque= b*(exp(u/-1.01)-1)/(-0.31)   ;
end

== matlab function draft7/L3/AR torque feedback L4/peacewise torque profile5 ==
  data: u input; torque output; a input; b input
function torque = T(u,a,b)    % Panjabi data fitted into logarithmic equation. Refer validation.xlsx
    torque = 0;
    if (u >= 0)
     torque= a*(exp(u/2.69)-1)/0.10;

    elseif (u < 0)
     torque= b*(exp(u/-0.90)-1)/(-0.89)   ;
end

== matlab function draft7/L3/FE torque feedback L4/peacewise torque profile1 ==
  data: u input; torque output; a input; b input

function torque = T(u,a,b)  % Guan et al logarithmic
    torque = 0;
    if (u >= 0)
     torque= a*(exp(u/11.09)-1)/0.09;

    elseif (u< 0)
     torque= b*(exp(u/-24.35)-1)/(-0.02)   ;
end

% function torque = T(u,a,b)  % Rao et al segmental
%     torque = 0;
%     if (u >= 0)
%         torque = (a)*(0.0342*u^3 + 0.0596*u^2 + 1.5861*u);
%     elseif (u< 0)
%         torque = (b)*(0.0342*u^3 + 0.0596*u^2 + 1.5861*u);
% end

== matlab function draft7/L3/LB torque feedback L4/peacewise torque profile4 ==
  data: u input; torque output; a input; b input
function torque = T(u,a,b)    % Guan et al (nonlinear logarithmic equation mentioned in their paper)
    torque = 0;
    if (u >= 0)
     torque= a*(exp(u/2.50)-1)/1.02;

    elseif (u< 0)
     torque= b*(exp(u/-2.58)-1)/(-0.82)   ;
end

== matlab function draft7/L2/AR torque feedback L4/peacewise torque profile5 ==
  data: u input; torque output; a input; b input
function torque = T(u,a,b)    % Panjabi data fitted into logarithmic equation. Refer validation.xlsx
    torque = 0;
    if (u >= 0)
     torque= a*(exp(u/0.80)-1)/0.93;

    elseif (u < 0)
     torque= b*(exp(u/-2.72)-1)/(-0.10)   ;
end
